simulink model "SDRE_controller"  (R2015a)
settings: Solver=ode45  StartTime=0.0  StopTime=10.0  RelTol=1e-3
undefined symbols (not defined in the file): m, n
settings Model: Creator=Amir  LastModifiedBy=Amir

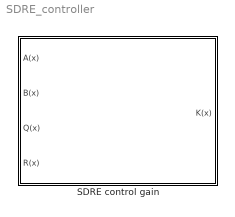
== system SDRE_controller ==
  SDRE control gain : Subsystem  mask{n=n, m=m}
      mask prompts: n "Length of state vector (x):"; m "Length of control input vector (u):"
      mask DialogControl DescGroupVar_copy Prompt: SDRE Controller
      mask DialogControl DescTextVar_copy_copy Prompt: This block calculates the controller obtained by the SDRE scheme.
      mask DialogControl DescGroupVar Prompt: System Dimension
      mask DialogControl Control4_copy_copy Prompt: 1- SDRE controller gain: K(x)
      mask DialogControl Control4_copy_copy_copy Prompt: Refer to the following link for the latest releases and more stuff about SDRE control technique:
      mask DialogControl Control8 Prompt: https://github.com/a-shakouri/SDRE_controller
      mask DialogControl Control8 Callback: web https://github.com/a-shakouri/SDRE_controller
      mask Display: fprintf('SDRE Controller')

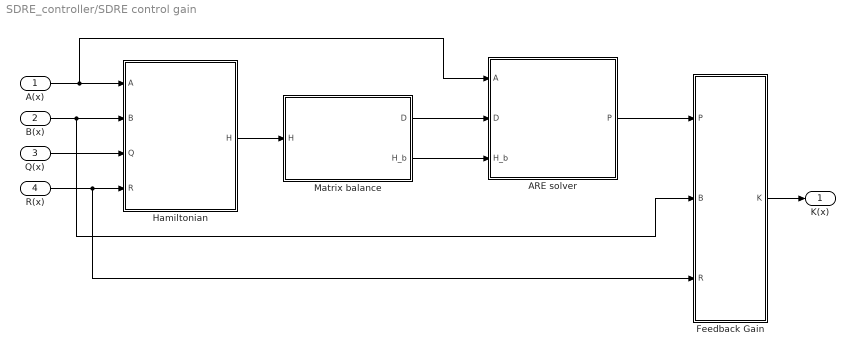
== system SDRE_controller/SDRE control gain ==
  A(x) : Inport
  B(x) : Inport  Port=2
  Q(x) : Inport  Port=3
  R(x) : Inport  Port=4
  ARE solver : MATLAB Function  TreatAsAtomicUnit=on
  Feedback Gain : MATLAB Function  TreatAsAtomicUnit=on
  Hamiltonian : MATLAB Function  TreatAsAtomicUnit=on
  Matrix balance : MATLAB Function  TreatAsAtomicUnit=on
  K(x) : Outport
  wires:
  Hamiltonian/1(H) -> Matrix balance/1(H)
  A(x)/1 -> Hamiltonian/1(A), ARE solver/1(A)
  Matrix balance/2(H_b) -> ARE solver/3(H_b)
  Matrix balance/1(D) -> ARE solver/2(D)
  ARE solver/1(P) -> Feedback Gain/1(P)
  B(x)/1 -> Feedback Gain/2(B), Hamiltonian/2(B)
  Feedback Gain/1(K) -> K(x)/1
  Q(x)/1 -> Hamiltonian/3(Q)
  R(x)/1 -> Feedback Gain/3(R), Hamiltonian/4(R)

== matlab function SDRE_controller/SDRE control gain/Hamiltonian ==
  data: A input size=[n n]; H output size=[2*n 2*n]; B input size=[n m]; Q input size=[n n]; R input size=[m m]
function H  = Hamilton(A, B, Q, R)
    
H = [A -(B/R)*B'; -Q -A'];

== matlab function SDRE_controller/SDRE control gain/Matrix balance ==
  data: H input size=[2*n 2*n]; D output size=[2*n 2*n]; H_b output size=[2*n 2*n]
function [D, H_b] = matrix_balance(H)
    
% Numerical Recipes p.593 - Balancing (vedi anche articolo James)
% Trasformazione
% D^-1 * A * D = B 
    
A=H;

    n = size(A,1);
    B = A;
    D = eye(n);
    
    RADIX = 2;
    sqrdx = RADIX*RADIX;
    
    done = 0;
    
    while done ~= 1 
        
        done = 1;
        
        for i = 1 : n 
            
            r = 0;
            c = 0;
            
            for j = 1 : n
                if j ~= i 
                    c = c + abs(B(j,i));
                    r = r + abs(B(i,j));
                end
            end
                
            if c ~= 0 && r ~= 0 
                g = r/RADIX;
                f = 1;
                s = c + r;
                
                while (c<g) 
                    f = f*RADIX;
                    c = c*sqrdx;
                end
                
                g = r*RADIX;
                
                while c > g 
                    f = f/RADIX;
                    c = c/sqrdx;
                end
                
                if (c + r)/f < 0.95*s 
                    done = 0;
                    g = 1/f;
                    D(i,i) = D(i,i)*f;

                    for j = 1 : n 
                        B(i,j) = B(i,j)/f; 
                    end
                    
                    for j = 1 : n
                        B(j,i) = B(j,i)*f;
                    end
                end
            end
        end
    end
    
H_b=B;

== matlab function SDRE_controller/SDRE control gain/ARE solver ==
  data: A input size=[n n]; D input size=[2*n 2*n]; H_b input size=[2*n 2*n]; P output size=[n n]
function P = ARE_diag(A, D, H_b)

    n = size(A,1);
    
    P = zeros(n,n);
    
    [T,L] = eig(H_b);
    
    T = D*T;
    
    lambda = diag(L);
    ord_lambda = zeros(1,2*n);
    for k = 1 : 2*n;
        if real(lambda(k)) < 0
            ord_lambda(k) = -1;
        elseif real(lambda(k)) > 0
            ord_lambda(k) = 1;
        else
            %disp('!!!');
        end
    end
    
    [~, ord_index] = sort(ord_lambda, 'descend');

    T_ord = T(:,ord_index);

    T22 = T_ord(n+1:2*n,n+1:2*n);
    T12 = T_ord(1:n,n+1:2*n);
    
    P = real(T22/T12);

== matlab function SDRE_controller/SDRE control gain/Feedback Gain ==
  data: P input size=[n n]; B input size=[n m]; K output size=[m n]; R input size=[m m]
function K  = u_in_gen(P,B,R)

K=-(inv(R))*B'*P;

end
